simulink model "elevatorMod"  (R2020a)
settings: Solver=VariableStepAuto  StartTime=0.0  StopTime=inf  RelTol=1e-3
PreLoadFcn:
  | slplc.api.loadDataTypes;
undefined symbols (not defined in the file): BOOL, DINT, INT, slplc
libraries: simulink x1
(part 28 of 39)

== system elevatorMod/PLCControllerSuite/__Logic/Task/Program/__Logic/XIC3/Instruction_Enable/__CoreVarRead ==
  DataRead : DataStoreRead  DataStoreName=xxx_PLC_VAR_F1PB
  y : Outport  VectorParamsAs1DForOutWhenUnconnected=off
  wires:
  DataRead/1 -> y/1

== system elevatorMod/PLCControllerSuite/__Logic/Task/Program/__Logic/XIC3/RungInOverride/ForceRungInFalseRead ==
  __CoreLabelRead : Subsystem  Tag=CoreVarReadBlock  DisableCoverage=on  TreatAsAtomicUnit=on  mask{PLCBlockType=CoreLabelRead}
      mask init:
      | slplc.callbacks.initRoutineLabelRead(gcb);
      mask Help: web([docroot '/plccoder/ref/__corelabelread' '.html']);
      mask DialogControl PLCBlockTitle Prompt: Core Label Read
  Out1 : Outport  VectorParamsAs1DForOutWhenUnconnected=off
  wires:
  __CoreLabelRead/1(Out1) -> Out1/1

== system elevatorMod/PLCControllerSuite/__Logic/Task/Program/__Logic/XIC30/BlockEnableRead/__CoreLabelRead ==
  DataRead : DataStoreRead  DataStoreName=x_PLCLabel__s4_3653__Block_Enable
  Out1 : Outport  VectorParamsAs1DForOutWhenUnconnected=off
  wires:
  DataRead/1 -> Out1/1

== system elevatorMod/PLCControllerSuite/__Logic/Task/Program/__Logic/XIC30/Instruction_Enable/__CoreVarRead ==
  DataRead : DataStoreRead  DataStoreName=xxx_PLC_VAR_F1PBHold
  y : Outport  VectorParamsAs1DForOutWhenUnconnected=off
  wires:
  DataRead/1 -> y/1

== system elevatorMod/PLCControllerSuite/__Logic/Task/Program/__Logic/XIC30/RungInOverride/ForceRungInFalseRead ==
  __CoreLabelRead : Subsystem  Tag=CoreVarReadBlock  DisableCoverage=on  TreatAsAtomicUnit=on  mask{PLCBlockType=CoreLabelRead}
      mask init:
      | slplc.callbacks.initRoutineLabelRead(gcb);
      mask Help: web([docroot '/plccoder/ref/__corelabelread' '.html']);
      mask DialogControl PLCBlockTitle Prompt: Core Label Read
  Out1 : Outport  VectorParamsAs1DForOutWhenUnconnected=off
  wires:
  __CoreLabelRead/1(Out1) -> Out1/1

== system elevatorMod/PLCControllerSuite/__Logic/Task/Program/__Logic/XIC31/BlockEnableRead/__CoreLabelRead ==
  DataRead : DataStoreRead  DataStoreName=x_PLCLabel__s4_3653__Block_Enable
  Out1 : Outport  VectorParamsAs1DForOutWhenUnconnected=off
  wires:
  DataRead/1 -> Out1/1

== system elevatorMod/PLCControllerSuite/__Logic/Task/Program/__Logic/XIC31/Instruction_Enable/__CoreVarRead ==
  DataRead : DataStoreRead  DataStoreName=xxx_PLC_VAR_StartHold
  y : Outport  VectorParamsAs1DForOutWhenUnconnected=off
  wires:
  DataRead/1 -> y/1

== system elevatorMod/PLCControllerSuite/__Logic/Task/Program/__Logic/XIC31/RungInOverride/ForceRungInFalseRead ==
  __CoreLabelRead : Subsystem  Tag=CoreVarReadBlock  DisableCoverage=on  TreatAsAtomicUnit=on  mask{PLCBlockType=CoreLabelRead}
      mask init:
      | slplc.callbacks.initRoutineLabelRead(gcb);
      mask Help: web([docroot '/plccoder/ref/__corelabelread' '.html']);
      mask DialogControl PLCBlockTitle Prompt: Core Label Read
  Out1 : Outport  VectorParamsAs1DForOutWhenUnconnected=off
  wires:
  __CoreLabelRead/1(Out1) -> Out1/1

== system elevatorMod/PLCControllerSuite/__Logic/Task/Program/__Logic/XIC32/BlockEnableRead/__CoreLabelRead ==
  DataRead : DataStoreRead  DataStoreName=x_PLCLabel__s4_3653__Block_Enable
  Out1 : Outport  VectorParamsAs1DForOutWhenUnconnected=off
  wires:
  DataRead/1 -> Out1/1

== system elevatorMod/PLCControllerSuite/__Logic/Task/Program/__Logic/XIC32/Instruction_Enable/__CoreVarRead ==
  DataRead : DataStoreRead  DataStoreName=xxx_PLC_VAR_LSTDIRUP
  y : Outport  VectorParamsAs1DForOutWhenUnconnected=off
  wires:
  DataRead/1 -> y/1

== system elevatorMod/PLCControllerSuite/__Logic/Task/Program/__Logic/XIC32/RungInOverride/ForceRungInFalseRead ==
  __CoreLabelRead : Subsystem  Tag=CoreVarReadBlock  DisableCoverage=on  TreatAsAtomicUnit=on  mask{PLCBlockType=CoreLabelRead}
      mask init:
      | slplc.callbacks.initRoutineLabelRead(gcb);
      mask Help: web([docroot '/plccoder/ref/__corelabelread' '.html']);
      mask DialogControl PLCBlockTitle Prompt: Core Label Read
  Out1 : Outport  VectorParamsAs1DForOutWhenUnconnected=off
  wires:
  __CoreLabelRead/1(Out1) -> Out1/1

== system elevatorMod/PLCControllerSuite/__Logic/Task/Program/__Logic/XIC33/BlockEnableRead/__CoreLabelRead ==
  DataRead : DataStoreRead  DataStoreName=x_PLCLabel__s4_3653__Block_Enable
  Out1 : Outport  VectorParamsAs1DForOutWhenUnconnected=off
  wires:
  DataRead/1 -> Out1/1

== system elevatorMod/PLCControllerSuite/__Logic/Task/Program/__Logic/XIC33/Instruction_Enable/__CoreVarRead ==
  DataRead : DataStoreRead  DataStoreName=xxx_PLC_VAR_GOINGUP
  y : Outport  VectorParamsAs1DForOutWhenUnconnected=off
  wires:
  DataRead/1 -> y/1

== system elevatorMod/PLCControllerSuite/__Logic/Task/Program/__Logic/XIC33/RungInOverride/ForceRungInFalseRead ==
  __CoreLabelRead : Subsystem  Tag=CoreVarReadBlock  DisableCoverage=on  TreatAsAtomicUnit=on  mask{PLCBlockType=CoreLabelRead}
      mask init:
      | slplc.callbacks.initRoutineLabelRead(gcb);
      mask Help: web([docroot '/plccoder/ref/__corelabelread' '.html']);
      mask DialogControl PLCBlockTitle Prompt: Core Label Read
  Out1 : Outport  VectorParamsAs1DForOutWhenUnconnected=off
  wires:
  __CoreLabelRead/1(Out1) -> Out1/1

== system elevatorMod/PLCControllerSuite/__Logic/Task/Program/__Logic/XIC34/BlockEnableRead/__CoreLabelRead ==
  DataRead : DataStoreRead  DataStoreName=x_PLCLabel__s4_3653__Block_Enable
  Out1 : Outport  VectorParamsAs1DForOutWhenUnconnected=off
  wires:
  DataRead/1 -> Out1/1

== system elevatorMod/PLCControllerSuite/__Logic/Task/Program/__Logic/XIC34/Instruction_Enable/__CoreVarRead ==
  DataRead : DataStoreRead  DataStoreName=xxx_PLC_VAR_MTRON
  y : Outport  VectorParamsAs1DForOutWhenUnconnected=off
  wires:
  DataRead/1 -> y/1

== system elevatorMod/PLCControllerSuite/__Logic/Task/Program/__Logic/XIC34/RungInOverride/ForceRungInFalseRead ==
  __CoreLabelRead : Subsystem  Tag=CoreVarReadBlock  DisableCoverage=on  TreatAsAtomicUnit=on  mask{PLCBlockType=CoreLabelRead}
      mask init:
      | slplc.callbacks.initRoutineLabelRead(gcb);
      mask Help: web([docroot '/plccoder/ref/__corelabelread' '.html']);
      mask DialogControl PLCBlockTitle Prompt: Core Label Read
  Out1 : Outport  VectorParamsAs1DForOutWhenUnconnected=off
  wires:
  __CoreLabelRead/1(Out1) -> Out1/1

== system elevatorMod/PLCControllerSuite/__Logic/Task/Program/__Logic/XIC35/BlockEnableRead/__CoreLabelRead ==
  DataRead : DataStoreRead  DataStoreName=x_PLCLabel__s4_3653__Block_Enable
  Out1 : Outport  VectorParamsAs1DForOutWhenUnconnected=off
  wires:
  DataRead/1 -> Out1/1

== system elevatorMod/PLCControllerSuite/__Logic/Task/Program/__Logic/XIC35/Instruction_Enable/__CoreVarRead ==
  DataRead : DataStoreRead  DataStoreName=xxx_PLC_VAR_F2PBHold
  y : Outport  VectorParamsAs1DForOutWhenUnconnected=off
  wires:
  DataRead/1 -> y/1

== system elevatorMod/PLCControllerSuite/__Logic/Task/Program/__Logic/XIC35/RungInOverride/ForceRungInFalseRead ==
  __CoreLabelRead : Subsystem  Tag=CoreVarReadBlock  DisableCoverage=on  TreatAsAtomicUnit=on  mask{PLCBlockType=CoreLabelRead}
      mask init:
      | slplc.callbacks.initRoutineLabelRead(gcb);
      mask Help: web([docroot '/plccoder/ref/__corelabelread' '.html']);
      mask DialogControl PLCBlockTitle Prompt: Core Label Read
  Out1 : Outport  VectorParamsAs1DForOutWhenUnconnected=off
  wires:
  __CoreLabelRead/1(Out1) -> Out1/1

== system elevatorMod/PLCControllerSuite/__Logic/Task/Program/__Logic/XIC36/BlockEnableRead/__CoreLabelRead ==
  DataRead : DataStoreRead  DataStoreName=x_PLCLabel__s4_3653__Block_Enable
  Out1 : Outport  VectorParamsAs1DForOutWhenUnconnected=off
  wires:
  DataRead/1 -> Out1/1

== system elevatorMod/PLCControllerSuite/__Logic/Task/Program/__Logic/XIC36/Instruction_Enable/__CoreVarRead ==
  DataRead : DataStoreRead  DataStoreName=xxx_PLC_VAR_F3DownBHold
  y : Outport  VectorParamsAs1DForOutWhenUnconnected=off
  wires:
  DataRead/1 -> y/1

== system elevatorMod/PLCControllerSuite/__Logic/Task/Program/__Logic/XIC36/RungInOverride/ForceRungInFalseRead ==
  __CoreLabelRead : Subsystem  Tag=CoreVarReadBlock  DisableCoverage=on  TreatAsAtomicUnit=on  mask{PLCBlockType=CoreLabelRead}
      mask init:
      | slplc.callbacks.initRoutineLabelRead(gcb);
      mask Help: web([docroot '/plccoder/ref/__corelabelread' '.html']);
      mask DialogControl PLCBlockTitle Prompt: Core Label Read
  Out1 : Outport  VectorParamsAs1DForOutWhenUnconnected=off
  wires:
  __CoreLabelRead/1(Out1) -> Out1/1

== system elevatorMod/PLCControllerSuite/__Logic/Task/Program/__Logic/XIC37/BlockEnableRead/__CoreLabelRead ==
  DataRead : DataStoreRead  DataStoreName=x_PLCLabel__s4_3653__Block_Enable
  Out1 : Outport  VectorParamsAs1DForOutWhenUnconnected=off
  wires:
  DataRead/1 -> Out1/1

== system elevatorMod/PLCControllerSuite/__Logic/Task/Program/__Logic/XIC37/Instruction_Enable/__CoreVarRead ==
  DataRead : DataStoreRead  DataStoreName=xxx_PLC_VAR_F2PBHold
  y : Outport  VectorParamsAs1DForOutWhenUnconnected=off
  wires:
  DataRead/1 -> y/1

== system elevatorMod/PLCControllerSuite/__Logic/Task/Program/__Logic/XIC37/RungInOverride/ForceRungInFalseRead ==
  __CoreLabelRead : Subsystem  Tag=CoreVarReadBlock  DisableCoverage=on  TreatAsAtomicUnit=on  mask{PLCBlockType=CoreLabelRead}
      mask init:
      | slplc.callbacks.initRoutineLabelRead(gcb);
      mask Help: web([docroot '/plccoder/ref/__corelabelread' '.html']);
      mask DialogControl PLCBlockTitle Prompt: Core Label Read
  Out1 : Outport  VectorParamsAs1DForOutWhenUnconnected=off
  wires:
  __CoreLabelRead/1(Out1) -> Out1/1

== system elevatorMod/PLCControllerSuite/__Logic/Task/Program/__Logic/XIC38/BlockEnableRead/__CoreLabelRead ==
  DataRead : DataStoreRead  DataStoreName=x_PLCLabel__s4_3653__Block_Enable
  Out1 : Outport  VectorParamsAs1DForOutWhenUnconnected=off
  wires:
  DataRead/1 -> Out1/1

== system elevatorMod/PLCControllerSuite/__Logic/Task/Program/__Logic/XIC38/Instruction_Enable/__CoreVarRead ==
  DataRead : DataStoreRead  DataStoreName=xxx_PLC_VAR_MTRON
  y : Outport  VectorParamsAs1DForOutWhenUnconnected=off
  wires:
  DataRead/1 -> y/1

== system elevatorMod/PLCControllerSuite/__Logic/Task/Program/__Logic/XIC38/RungInOverride/ForceRungInFalseRead ==
  __CoreLabelRead : Subsystem  Tag=CoreVarReadBlock  DisableCoverage=on  TreatAsAtomicUnit=on  mask{PLCBlockType=CoreLabelRead}
      mask init:
      | slplc.callbacks.initRoutineLabelRead(gcb);
      mask Help: web([docroot '/plccoder/ref/__corelabelread' '.html']);
      mask DialogControl PLCBlockTitle Prompt: Core Label Read
  Out1 : Outport  VectorParamsAs1DForOutWhenUnconnected=off
  wires:
  __CoreLabelRead/1(Out1) -> Out1/1

== system elevatorMod/PLCControllerSuite/__Logic/Task/Program/__Logic/XIC39/BlockEnableRead/__CoreLabelRead ==
  DataRead : DataStoreRead  DataStoreName=x_PLCLabel__s4_3653__Block_Enable
  Out1 : Outport  VectorParamsAs1DForOutWhenUnconnected=off
  wires:
  DataRead/1 -> Out1/1

== system elevatorMod/PLCControllerSuite/__Logic/Task/Program/__Logic/XIC39/Instruction_Enable/__CoreVarRead ==
  DataRead : DataStoreRead  DataStoreName=xxx_PLC_VAR_RMPUPTRG
  y : Outport  VectorParamsAs1DForOutWhenUnconnected=off
  wires:
  DataRead/1 -> y/1

== system elevatorMod/PLCControllerSuite/__Logic/Task/Program/__Logic/XIC39/RungInOverride/ForceRungInFalseRead ==
  __CoreLabelRead : Subsystem  Tag=CoreVarReadBlock  DisableCoverage=on  TreatAsAtomicUnit=on  mask{PLCBlockType=CoreLabelRead}
      mask init:
      | slplc.callbacks.initRoutineLabelRead(gcb);
      mask Help: web([docroot '/plccoder/ref/__corelabelread' '.html']);
      mask DialogControl PLCBlockTitle Prompt: Core Label Read
  Out1 : Outport  VectorParamsAs1DForOutWhenUnconnected=off
  wires:
  __CoreLabelRead/1(Out1) -> Out1/1

== system elevatorMod/PLCControllerSuite/__Logic/Task/Program/__Logic/XIC4/BlockEnableRead/__CoreLabelRead ==
  DataRead : DataStoreRead  DataStoreName=x_PLCLabel__s4_3653__Block_Enable
  Out1 : Outport  VectorParamsAs1DForOutWhenUnconnected=off
  wires:
  DataRead/1 -> Out1/1

== system elevatorMod/PLCControllerSuite/__Logic/Task/Program/__Logic/XIC4/Instruction_Enable/__CoreVarRead ==
  DataRead : DataStoreRead  DataStoreName=xxx_PLC_VAR_F1PBHold
  y : Outport  VectorParamsAs1DForOutWhenUnconnected=off
  wires:
  DataRead/1 -> y/1

== system elevatorMod/PLCControllerSuite/__Logic/Task/Program/__Logic/XIC4/RungInOverride/ForceRungInFalseRead ==
  __CoreLabelRead : Subsystem  Tag=CoreVarReadBlock  DisableCoverage=on  TreatAsAtomicUnit=on  mask{PLCBlockType=CoreLabelRead}
      mask init:
      | slplc.callbacks.initRoutineLabelRead(gcb);
      mask Help: web([docroot '/plccoder/ref/__corelabelread' '.html']);
      mask DialogControl PLCBlockTitle Prompt: Core Label Read
  Out1 : Outport  VectorParamsAs1DForOutWhenUnconnected=off
  wires:
  __CoreLabelRead/1(Out1) -> Out1/1

== system elevatorMod/PLCControllerSuite/__Logic/Task/Program/__Logic/XIC40/BlockEnableRead/__CoreLabelRead ==
  DataRead : DataStoreRead  DataStoreName=x_PLCLabel__s4_3653__Block_Enable
  Out1 : Outport  VectorParamsAs1DForOutWhenUnconnected=off
  wires:
  DataRead/1 -> Out1/1

== system elevatorMod/PLCControllerSuite/__Logic/Task/Program/__Logic/XIC40/Instruction_Enable/__CoreVarRead ==
  DataRead : DataStoreRead  DataStoreName=xxx_PLC_VAR_RMPUP
  y : Outport  VectorParamsAs1DForOutWhenUnconnected=off
  wires:
  DataRead/1 -> y/1

== system elevatorMod/PLCControllerSuite/__Logic/Task/Program/__Logic/XIC40/RungInOverride/ForceRungInFalseRead ==
  __CoreLabelRead : Subsystem  Tag=CoreVarReadBlock  DisableCoverage=on  TreatAsAtomicUnit=on  mask{PLCBlockType=CoreLabelRead}
      mask init:
      | slplc.callbacks.initRoutineLabelRead(gcb);
      mask Help: web([docroot '/plccoder/ref/__corelabelread' '.html']);
      mask DialogControl PLCBlockTitle Prompt: Core Label Read
  Out1 : Outport  VectorParamsAs1DForOutWhenUnconnected=off
  wires:
  __CoreLabelRead/1(Out1) -> Out1/1

== system elevatorMod/PLCControllerSuite/__Logic/Task/Program/__Logic/XIC41/BlockEnableRead/__CoreLabelRead ==
  DataRead : DataStoreRead  DataStoreName=x_PLCLabel__s4_3653__Block_Enable
  Out1 : Outport  VectorParamsAs1DForOutWhenUnconnected=off
  wires:
  DataRead/1 -> Out1/1

== system elevatorMod/PLCControllerSuite/__Logic/Task/Program/__Logic/XIC41/Instruction_Enable/__CoreVarRead ==
  DataRead : DataStoreRead  DataStoreName=xxx_PLC_VAR_SENCHK
  y : Outport  VectorParamsAs1DForOutWhenUnconnected=off
  wires:
  DataRead/1 -> y/1

== system elevatorMod/PLCControllerSuite/__Logic/Task/Program/__Logic/XIC41/RungInOverride/ForceRungInFalseRead ==
  __CoreLabelRead : Subsystem  Tag=CoreVarReadBlock  DisableCoverage=on  TreatAsAtomicUnit=on  mask{PLCBlockType=CoreLabelRead}
      mask init:
      | slplc.callbacks.initRoutineLabelRead(gcb);
      mask Help: web([docroot '/plccoder/ref/__corelabelread' '.html']);
      mask DialogControl PLCBlockTitle Prompt: Core Label Read
  Out1 : Outport  VectorParamsAs1DForOutWhenUnconnected=off
  wires:
  __CoreLabelRead/1(Out1) -> Out1/1

== system elevatorMod/PLCControllerSuite/__Logic/Task/Program/__Logic/XIC42/BlockEnableRead/__CoreLabelRead ==
  DataRead : DataStoreRead  DataStoreName=x_PLCLabel__s4_3653__Block_Enable
  Out1 : Outport  VectorParamsAs1DForOutWhenUnconnected=off
  wires:
  DataRead/1 -> Out1/1

== system elevatorMod/PLCControllerSuite/__Logic/Task/Program/__Logic/XIC42/Instruction_Enable/__CoreVarRead ==
  DataRead : DataStoreRead  DataStoreName=xxx_PLC_VAR_StartHold
  y : Outport  VectorParamsAs1DForOutWhenUnconnected=off
  wires:
  DataRead/1 -> y/1

== system elevatorMod/PLCControllerSuite/__Logic/Task/Program/__Logic/XIC42/RungInOverride/ForceRungInFalseRead ==
  __CoreLabelRead : Subsystem  Tag=CoreVarReadBlock  DisableCoverage=on  TreatAsAtomicUnit=on  mask{PLCBlockType=CoreLabelRead}
      mask init:
      | slplc.callbacks.initRoutineLabelRead(gcb);
      mask Help: web([docroot '/plccoder/ref/__corelabelread' '.html']);
      mask DialogControl PLCBlockTitle Prompt: Core Label Read
  Out1 : Outport  VectorParamsAs1DForOutWhenUnconnected=off
  wires:
  __CoreLabelRead/1(Out1) -> Out1/1

== system elevatorMod/PLCControllerSuite/__Logic/Task/Program/__Logic/XIC43/BlockEnableRead/__CoreLabelRead ==
  DataRead : DataStoreRead  DataStoreName=x_PLCLabel__s4_3653__Block_Enable
  Out1 : Outport  VectorParamsAs1DForOutWhenUnconnected=off
  wires:
  DataRead/1 -> Out1/1

== system elevatorMod/PLCControllerSuite/__Logic/Task/Program/__Logic/XIC43/Instruction_Enable/__CoreVarRead ==
  DataRead : DataStoreRead  DataStoreName=xxx_PLC_VAR_TempS3LUp
  y : Outport  VectorParamsAs1DForOutWhenUnconnected=off
  wires:
  DataRead/1 -> y/1

== system elevatorMod/PLCControllerSuite/__Logic/Task/Program/__Logic/XIC43/RungInOverride/ForceRungInFalseRead ==
  __CoreLabelRead : Subsystem  Tag=CoreVarReadBlock  DisableCoverage=on  TreatAsAtomicUnit=on  mask{PLCBlockType=CoreLabelRead}
      mask init:
      | slplc.callbacks.initRoutineLabelRead(gcb);
      mask Help: web([docroot '/plccoder/ref/__corelabelread' '.html']);
      mask DialogControl PLCBlockTitle Prompt: Core Label Read
  Out1 : Outport  VectorParamsAs1DForOutWhenUnconnected=off
  wires:
  __CoreLabelRead/1(Out1) -> Out1/1

== system elevatorMod/PLCControllerSuite/__Logic/Task/Program/__Logic/XIC44/BlockEnableRead/__CoreLabelRead ==
  DataRead : DataStoreRead  DataStoreName=x_PLCLabel__s4_3653__Block_Enable
  Out1 : Outport  VectorParamsAs1DForOutWhenUnconnected=off
  wires:
  DataRead/1 -> Out1/1

== system elevatorMod/PLCControllerSuite/__Logic/Task/Program/__Logic/XIC44/Instruction_Enable/__CoreVarRead ==
  DataRead : DataStoreRead  DataStoreName=xxx_PLC_VAR_MemoryGoUp
  y : Outport  VectorParamsAs1DForOutWhenUnconnected=off
  wires:
  DataRead/1 -> y/1

== system elevatorMod/PLCControllerSuite/__Logic/Task/Program/__Logic/XIC44/RungInOverride/ForceRungInFalseRead ==
  __CoreLabelRead : Subsystem  Tag=CoreVarReadBlock  DisableCoverage=on  TreatAsAtomicUnit=on  mask{PLCBlockType=CoreLabelRead}
      mask init:
      | slplc.callbacks.initRoutineLabelRead(gcb);
      mask Help: web([docroot '/plccoder/ref/__corelabelread' '.html']);
      mask DialogControl PLCBlockTitle Prompt: Core Label Read
  Out1 : Outport  VectorParamsAs1DForOutWhenUnconnected=off
  wires:
  __CoreLabelRead/1(Out1) -> Out1/1

== system elevatorMod/PLCControllerSuite/__Logic/Task/Program/__Logic/XIC45/BlockEnableRead/__CoreLabelRead ==
  DataRead : DataStoreRead  DataStoreName=x_PLCLabel__s4_3653__Block_Enable
  Out1 : Outport  VectorParamsAs1DForOutWhenUnconnected=off
  wires:
  DataRead/1 -> Out1/1

== system elevatorMod/PLCControllerSuite/__Logic/Task/Program/__Logic/XIC45/Instruction_Enable/__CoreVarRead ==
  DataRead : DataStoreRead  DataStoreName=xxx_PLC_VAR_StartHold
  y : Outport  VectorParamsAs1DForOutWhenUnconnected=off
  wires:
  DataRead/1 -> y/1

== system elevatorMod/PLCControllerSuite/__Logic/Task/Program/__Logic/XIC45/RungInOverride/ForceRungInFalseRead ==
  __CoreLabelRead : Subsystem  Tag=CoreVarReadBlock  DisableCoverage=on  TreatAsAtomicUnit=on  mask{PLCBlockType=CoreLabelRead}
      mask init:
      | slplc.callbacks.initRoutineLabelRead(gcb);
      mask Help: web([docroot '/plccoder/ref/__corelabelread' '.html']);
      mask DialogControl PLCBlockTitle Prompt: Core Label Read
  Out1 : Outport  VectorParamsAs1DForOutWhenUnconnected=off
  wires:
  __CoreLabelRead/1(Out1) -> Out1/1

== system elevatorMod/PLCControllerSuite/__Logic/Task/Program/__Logic/XIC46/BlockEnableRead/__CoreLabelRead ==
  DataRead : DataStoreRead  DataStoreName=x_PLCLabel__s4_3653__Block_Enable
  Out1 : Outport  VectorParamsAs1DForOutWhenUnconnected=off
  wires:
  DataRead/1 -> Out1/1

== system elevatorMod/PLCControllerSuite/__Logic/Task/Program/__Logic/XIC46/Instruction_Enable/__CoreVarRead ==
  DataRead : DataStoreRead  DataStoreName=xxx_PLC_VAR_S1H
  y : Outport  VectorParamsAs1DForOutWhenUnconnected=off
  wires:
  DataRead/1 -> y/1

== system elevatorMod/PLCControllerSuite/__Logic/Task/Program/__Logic/XIC46/RungInOverride/ForceRungInFalseRead ==
  __CoreLabelRead : Subsystem  Tag=CoreVarReadBlock  DisableCoverage=on  TreatAsAtomicUnit=on  mask{PLCBlockType=CoreLabelRead}
      mask init:
      | slplc.callbacks.initRoutineLabelRead(gcb);
      mask Help: web([docroot '/plccoder/ref/__corelabelread' '.html']);
      mask DialogControl PLCBlockTitle Prompt: Core Label Read
  Out1 : Outport  VectorParamsAs1DForOutWhenUnconnected=off
  wires:
  __CoreLabelRead/1(Out1) -> Out1/1

== system elevatorMod/PLCControllerSuite/__Logic/Task/Program/__Logic/XIC47/BlockEnableRead/__CoreLabelRead ==
  DataRead : DataStoreRead  DataStoreName=x_PLCLabel__s4_3653__Block_Enable
  Out1 : Outport  VectorParamsAs1DForOutWhenUnconnected=off
  wires:
  DataRead/1 -> Out1/1

== system elevatorMod/PLCControllerSuite/__Logic/Task/Program/__Logic/XIC47/Instruction_Enable/__CoreVarRead ==
  DataRead : DataStoreRead  DataStoreName=xxx_PLC_VAR_S2L
  y : Outport  VectorParamsAs1DForOutWhenUnconnected=off
  wires:
  DataRead/1 -> y/1

== system elevatorMod/PLCControllerSuite/__Logic/Task/Program/__Logic/XIC47/RungInOverride/ForceRungInFalseRead ==
  __CoreLabelRead : Subsystem  Tag=CoreVarReadBlock  DisableCoverage=on  TreatAsAtomicUnit=on  mask{PLCBlockType=CoreLabelRead}
      mask init:
      | slplc.callbacks.initRoutineLabelRead(gcb);
      mask Help: web([docroot '/plccoder/ref/__corelabelread' '.html']);
      mask DialogControl PLCBlockTitle Prompt: Core Label Read
  Out1 : Outport  VectorParamsAs1DForOutWhenUnconnected=off
  wires:
  __CoreLabelRead/1(Out1) -> Out1/1

== system elevatorMod/PLCControllerSuite/__Logic/Task/Program/__Logic/XIC48/BlockEnableRead/__CoreLabelRead ==
  DataRead : DataStoreRead  DataStoreName=x_PLCLabel__s4_3653__Block_Enable
  Out1 : Outport  VectorParamsAs1DForOutWhenUnconnected=off
  wires:
  DataRead/1 -> Out1/1

== system elevatorMod/PLCControllerSuite/__Logic/Task/Program/__Logic/XIC48/Instruction_Enable/__CoreVarRead ==
  DataRead : DataStoreRead  DataStoreName=xxx_PLC_VAR_F2UpDownBHold
  y : Outport  VectorParamsAs1DForOutWhenUnconnected=off
  wires:
  DataRead/1 -> y/1

== system elevatorMod/PLCControllerSuite/__Logic/Task/Program/__Logic/XIC48/RungInOverride/ForceRungInFalseRead ==
  __CoreLabelRead : Subsystem  Tag=CoreVarReadBlock  DisableCoverage=on  TreatAsAtomicUnit=on  mask{PLCBlockType=CoreLabelRead}
      mask init:
      | slplc.callbacks.initRoutineLabelRead(gcb);
      mask Help: web([docroot '/plccoder/ref/__corelabelread' '.html']);
      mask DialogControl PLCBlockTitle Prompt: Core Label Read
  Out1 : Outport  VectorParamsAs1DForOutWhenUnconnected=off
  wires:
  __CoreLabelRead/1(Out1) -> Out1/1

== system elevatorMod/PLCControllerSuite/__Logic/Task/Program/__Logic/XIC49/BlockEnableRead/__CoreLabelRead ==
  DataRead : DataStoreRead  DataStoreName=x_PLCLabel__s4_3653__Block_Enable
  Out1 : Outport  VectorParamsAs1DForOutWhenUnconnected=off
  wires:
  DataRead/1 -> Out1/1

== system elevatorMod/PLCControllerSuite/__Logic/Task/Program/__Logic/XIC49/Instruction_Enable/__CoreVarRead ==
  DataRead : DataStoreRead  DataStoreName=xxx_PLC_VAR_S3L
  y : Outport  VectorParamsAs1DForOutWhenUnconnected=off
  wires:
  DataRead/1 -> y/1

== system elevatorMod/PLCControllerSuite/__Logic/Task/Program/__Logic/XIC49/RungInOverride/ForceRungInFalseRead ==
  __CoreLabelRead : Subsystem  Tag=CoreVarReadBlock  DisableCoverage=on  TreatAsAtomicUnit=on  mask{PLCBlockType=CoreLabelRead}
      mask init:
      | slplc.callbacks.initRoutineLabelRead(gcb);
      mask Help: web([docroot '/plccoder/ref/__corelabelread' '.html']);
      mask DialogControl PLCBlockTitle Prompt: Core Label Read
  Out1 : Outport  VectorParamsAs1DForOutWhenUnconnected=off
  wires:
  __CoreLabelRead/1(Out1) -> Out1/1

== system elevatorMod/PLCControllerSuite/__Logic/Task/Program/__Logic/XIC5/BlockEnableRead/__CoreLabelRead ==
  DataRead : DataStoreRead  DataStoreName=x_PLCLabel__s4_3653__Block_Enable
  Out1 : Outport  VectorParamsAs1DForOutWhenUnconnected=off
  wires:
  DataRead/1 -> Out1/1

== system elevatorMod/PLCControllerSuite/__Logic/Task/Program/__Logic/XIC5/Instruction_Enable/__CoreVarRead ==
  DataRead : DataStoreRead  DataStoreName=xxx_PLC_VAR_StartHold
  y : Outport  VectorParamsAs1DForOutWhenUnconnected=off
  wires:
  DataRead/1 -> y/1

== system elevatorMod/PLCControllerSuite/__Logic/Task/Program/__Logic/XIC5/RungInOverride/ForceRungInFalseRead ==
  __CoreLabelRead : Subsystem  Tag=CoreVarReadBlock  DisableCoverage=on  TreatAsAtomicUnit=on  mask{PLCBlockType=CoreLabelRead}
      mask init:
      | slplc.callbacks.initRoutineLabelRead(gcb);
      mask Help: web([docroot '/plccoder/ref/__corelabelread' '.html']);
      mask DialogControl PLCBlockTitle Prompt: Core Label Read
  Out1 : Outport  VectorParamsAs1DForOutWhenUnconnected=off
  wires:
  __CoreLabelRead/1(Out1) -> Out1/1

== system elevatorMod/PLCControllerSuite/__Logic/Task/Program/__Logic/XIC50/BlockEnableRead/__CoreLabelRead ==
  DataRead : DataStoreRead  DataStoreName=x_PLCLabel__s4_3653__Block_Enable
  Out1 : Outport  VectorParamsAs1DForOutWhenUnconnected=off
  wires:
  DataRead/1 -> Out1/1

== system elevatorMod/PLCControllerSuite/__Logic/Task/Program/__Logic/XIC50/Instruction_Enable/__CoreVarRead ==
  DataRead : DataStoreRead  DataStoreName=xxx_PLC_VAR_S2H
  y : Outport  VectorParamsAs1DForOutWhenUnconnected=off
  wires:
  DataRead/1 -> y/1

== system elevatorMod/PLCControllerSuite/__Logic/Task/Program/__Logic/XIC50/RungInOverride/ForceRungInFalseRead ==
  __CoreLabelRead : Subsystem  Tag=CoreVarReadBlock  DisableCoverage=on  TreatAsAtomicUnit=on  mask{PLCBlockType=CoreLabelRead}
      mask init:
      | slplc.callbacks.initRoutineLabelRead(gcb);
      mask Help: web([docroot '/plccoder/ref/__corelabelread' '.html']);
      mask DialogControl PLCBlockTitle Prompt: Core Label Read
  Out1 : Outport  VectorParamsAs1DForOutWhenUnconnected=off
  wires:
  __CoreLabelRead/1(Out1) -> Out1/1

== system elevatorMod/PLCControllerSuite/__Logic/Task/Program/__Logic/XIC51/BlockEnableRead/__CoreLabelRead ==
  DataRead : DataStoreRead  DataStoreName=x_PLCLabel__s4_3653__Block_Enable
  Out1 : Outport  VectorParamsAs1DForOutWhenUnconnected=off
  wires:
  DataRead/1 -> Out1/1

== system elevatorMod/PLCControllerSuite/__Logic/Task/Program/__Logic/XIC51/Instruction_Enable/__CoreVarRead ==
  DataRead : DataStoreRead  DataStoreName=xxx_PLC_VAR_F1PBHold
  y : Outport  VectorParamsAs1DForOutWhenUnconnected=off
  wires:
  DataRead/1 -> y/1

== system elevatorMod/PLCControllerSuite/__Logic/Task/Program/__Logic/XIC51/RungInOverride/ForceRungInFalseRead ==
  __CoreLabelRead : Subsystem  Tag=CoreVarReadBlock  DisableCoverage=on  TreatAsAtomicUnit=on  mask{PLCBlockType=CoreLabelRead}
      mask init:
      | slplc.callbacks.initRoutineLabelRead(gcb);
      mask Help: web([docroot '/plccoder/ref/__corelabelread' '.html']);
      mask DialogControl PLCBlockTitle Prompt: Core Label Read
  Out1 : Outport  VectorParamsAs1DForOutWhenUnconnected=off
  wires:
  __CoreLabelRead/1(Out1) -> Out1/1

== system elevatorMod/PLCControllerSuite/__Logic/Task/Program/__Logic/XIC52/BlockEnableRead/__CoreLabelRead ==
  DataRead : DataStoreRead  DataStoreName=x_PLCLabel__s4_3653__Block_Enable
  Out1 : Outport  VectorParamsAs1DForOutWhenUnconnected=off
  wires:
  DataRead/1 -> Out1/1

== system elevatorMod/PLCControllerSuite/__Logic/Task/Program/__Logic/XIC52/Instruction_Enable/__CoreVarRead ==
  DataRead : DataStoreRead  DataStoreName=xxx_PLC_VAR_F2UpDownBHold
  y : Outport  VectorParamsAs1DForOutWhenUnconnected=off
  wires:
  DataRead/1 -> y/1

== system elevatorMod/PLCControllerSuite/__Logic/Task/Program/__Logic/XIC52/RungInOverride/ForceRungInFalseRead ==
  __CoreLabelRead : Subsystem  Tag=CoreVarReadBlock  DisableCoverage=on  TreatAsAtomicUnit=on  mask{PLCBlockType=CoreLabelRead}
      mask init:
      | slplc.callbacks.initRoutineLabelRead(gcb);
      mask Help: web([docroot '/plccoder/ref/__corelabelread' '.html']);
      mask DialogControl PLCBlockTitle Prompt: Core Label Read
  Out1 : Outport  VectorParamsAs1DForOutWhenUnconnected=off
  wires:
  __CoreLabelRead/1(Out1) -> Out1/1

== system elevatorMod/PLCControllerSuite/__Logic/Task/Program/__Logic/XIC53/BlockEnableRead/__CoreLabelRead ==
  DataRead : DataStoreRead  DataStoreName=x_PLCLabel__s4_3653__Block_Enable
  Out1 : Outport  VectorParamsAs1DForOutWhenUnconnected=off
  wires:
  DataRead/1 -> Out1/1

== system elevatorMod/PLCControllerSuite/__Logic/Task/Program/__Logic/XIC53/Instruction_Enable/__CoreVarRead ==
  DataRead : DataStoreRead  DataStoreName=xxx_PLC_VAR_GOINGUP
  y : Outport  VectorParamsAs1DForOutWhenUnconnected=off
  wires:
  DataRead/1 -> y/1

== system elevatorMod/PLCControllerSuite/__Logic/Task/Program/__Logic/XIC53/RungInOverride/ForceRungInFalseRead ==
  __CoreLabelRead : Subsystem  Tag=CoreVarReadBlock  DisableCoverage=on  TreatAsAtomicUnit=on  mask{PLCBlockType=CoreLabelRead}
      mask init:
      | slplc.callbacks.initRoutineLabelRead(gcb);
      mask Help: web([docroot '/plccoder/ref/__corelabelread' '.html']);
      mask DialogControl PLCBlockTitle Prompt: Core Label Read
  Out1 : Outport  VectorParamsAs1DForOutWhenUnconnected=off
  wires:
  __CoreLabelRead/1(Out1) -> Out1/1

== system elevatorMod/PLCControllerSuite/__Logic/Task/Program/__Logic/XIC54/BlockEnableRead/__CoreLabelRead ==
  DataRead : DataStoreRead  DataStoreName=x_PLCLabel__s4_3653__Block_Enable
  Out1 : Outport  VectorParamsAs1DForOutWhenUnconnected=off
  wires:
  DataRead/1 -> Out1/1

== system elevatorMod/PLCControllerSuite/__Logic/Task/Program/__Logic/XIC54/Instruction_Enable/__CoreVarRead ==
  DataRead : DataStoreRead  DataStoreName=xxx_PLC_VAR_F3PBHold
  y : Outport  VectorParamsAs1DForOutWhenUnconnected=off
  wires:
  DataRead/1 -> y/1

== system elevatorMod/PLCControllerSuite/__Logic/Task/Program/__Logic/XIC54/RungInOverride/ForceRungInFalseRead ==
  __CoreLabelRead : Subsystem  Tag=CoreVarReadBlock  DisableCoverage=on  TreatAsAtomicUnit=on  mask{PLCBlockType=CoreLabelRead}
      mask init:
      | slplc.callbacks.initRoutineLabelRead(gcb);
      mask Help: web([docroot '/plccoder/ref/__corelabelread' '.html']);
      mask DialogControl PLCBlockTitle Prompt: Core Label Read
  Out1 : Outport  VectorParamsAs1DForOutWhenUnconnected=off
  wires:
  __CoreLabelRead/1(Out1) -> Out1/1

== system elevatorMod/PLCControllerSuite/__Logic/Task/Program/__Logic/XIC55/BlockEnableRead/__CoreLabelRead ==
  DataRead : DataStoreRead  DataStoreName=x_PLCLabel__s4_3653__Block_Enable
  Out1 : Outport  VectorParamsAs1DForOutWhenUnconnected=off
  wires:
  DataRead/1 -> Out1/1

== system elevatorMod/PLCControllerSuite/__Logic/Task/Program/__Logic/XIC55/Instruction_Enable/__CoreVarRead ==
  DataRead : DataStoreRead  DataStoreName=xxx_PLC_VAR_GOINGDN
  y : Outport  VectorParamsAs1DForOutWhenUnconnected=off
  wires:
  DataRead/1 -> y/1

== system elevatorMod/PLCControllerSuite/__Logic/Task/Program/__Logic/XIC55/RungInOverride/ForceRungInFalseRead ==
  __CoreLabelRead : Subsystem  Tag=CoreVarReadBlock  DisableCoverage=on  TreatAsAtomicUnit=on  mask{PLCBlockType=CoreLabelRead}
      mask init:
      | slplc.callbacks.initRoutineLabelRead(gcb);
      mask Help: web([docroot '/plccoder/ref/__corelabelread' '.html']);
      mask DialogControl PLCBlockTitle Prompt: Core Label Read
  Out1 : Outport  VectorParamsAs1DForOutWhenUnconnected=off
  wires:
  __CoreLabelRead/1(Out1) -> Out1/1

== system elevatorMod/PLCControllerSuite/__Logic/Task/Program/__Logic/XIC56/BlockEnableRead/__CoreLabelRead ==
  DataRead : DataStoreRead  DataStoreName=x_PLCLabel__s4_3653__Block_Enable
  Out1 : Outport  VectorParamsAs1DForOutWhenUnconnected=off
  wires:
  DataRead/1 -> Out1/1

== system elevatorMod/PLCControllerSuite/__Logic/Task/Program/__Logic/XIC56/Instruction_Enable/__CoreVarRead ==
  DataRead : DataStoreRead  DataStoreName=xxx_PLC_VAR_StartHold
  y : Outport  VectorParamsAs1DForOutWhenUnconnected=off
  wires:
  DataRead/1 -> y/1

== system elevatorMod/PLCControllerSuite/__Logic/Task/Program/__Logic/XIC56/RungInOverride/ForceRungInFalseRead ==
  __CoreLabelRead : Subsystem  Tag=CoreVarReadBlock  DisableCoverage=on  TreatAsAtomicUnit=on  mask{PLCBlockType=CoreLabelRead}
      mask init:
      | slplc.callbacks.initRoutineLabelRead(gcb);
      mask Help: web([docroot '/plccoder/ref/__corelabelread' '.html']);
      mask DialogControl PLCBlockTitle Prompt: Core Label Read
  Out1 : Outport  VectorParamsAs1DForOutWhenUnconnected=off
  wires:
  __CoreLabelRead/1(Out1) -> Out1/1

== system elevatorMod/PLCControllerSuite/__Logic/Task/Program/__Logic/XIC57/BlockEnableRead/__CoreLabelRead ==
  DataRead : DataStoreRead  DataStoreName=x_PLCLabel__s4_3653__Block_Enable
  Out1 : Outport  VectorParamsAs1DForOutWhenUnconnected=off
  wires:
  DataRead/1 -> Out1/1

== system elevatorMod/PLCControllerSuite/__Logic/Task/Program/__Logic/XIC57/Instruction_Enable/__CoreVarRead ==
  DataRead : DataStoreRead  DataStoreName=xxx_PLC_VAR_F1UpBHold
  y : Outport  VectorParamsAs1DForOutWhenUnconnected=off
  wires:
  DataRead/1 -> y/1

== system elevatorMod/PLCControllerSuite/__Logic/Task/Program/__Logic/XIC57/RungInOverride/ForceRungInFalseRead ==
  __CoreLabelRead : Subsystem  Tag=CoreVarReadBlock  DisableCoverage=on  TreatAsAtomicUnit=on  mask{PLCBlockType=CoreLabelRead}
      mask init:
      | slplc.callbacks.initRoutineLabelRead(gcb);
      mask Help: web([docroot '/plccoder/ref/__corelabelread' '.html']);
      mask DialogControl PLCBlockTitle Prompt: Core Label Read
  Out1 : Outport  VectorParamsAs1DForOutWhenUnconnected=off
  wires:
  __CoreLabelRead/1(Out1) -> Out1/1

== system elevatorMod/PLCControllerSuite/__Logic/Task/Program/__Logic/XIC58/BlockEnableRead/__CoreLabelRead ==
  DataRead : DataStoreRead  DataStoreName=x_PLCLabel__s4_3653__Block_Enable
  Out1 : Outport  VectorParamsAs1DForOutWhenUnconnected=off
  wires:
  DataRead/1 -> Out1/1

== system elevatorMod/PLCControllerSuite/__Logic/Task/Program/__Logic/XIC58/Instruction_Enable/__CoreVarRead ==
  DataRead : DataStoreRead  DataStoreName=xxx_PLC_VAR_StartHold
  y : Outport  VectorParamsAs1DForOutWhenUnconnected=off
  wires:
  DataRead/1 -> y/1

== system elevatorMod/PLCControllerSuite/__Logic/Task/Program/__Logic/XIC58/RungInOverride/ForceRungInFalseRead ==
  __CoreLabelRead : Subsystem  Tag=CoreVarReadBlock  DisableCoverage=on  TreatAsAtomicUnit=on  mask{PLCBlockType=CoreLabelRead}
      mask init:
      | slplc.callbacks.initRoutineLabelRead(gcb);
      mask Help: web([docroot '/plccoder/ref/__corelabelread' '.html']);
      mask DialogControl PLCBlockTitle Prompt: Core Label Read
  Out1 : Outport  VectorParamsAs1DForOutWhenUnconnected=off
  wires:
  __CoreLabelRead/1(Out1) -> Out1/1

== system elevatorMod/PLCControllerSuite/__Logic/Task/Program/__Logic/XIC59/BlockEnableRead/__CoreLabelRead ==
  DataRead : DataStoreRead  DataStoreName=x_PLCLabel__s4_3653__Block_Enable
  Out1 : Outport  VectorParamsAs1DForOutWhenUnconnected=off
  wires:
  DataRead/1 -> Out1/1

== system elevatorMod/PLCControllerSuite/__Logic/Task/Program/__Logic/XIC59/Instruction_Enable/__CoreVarRead ==
  DataRead : DataStoreRead  DataStoreName=xxx_PLC_VAR_StartHold
  y : Outport  VectorParamsAs1DForOutWhenUnconnected=off
  wires:
  DataRead/1 -> y/1

== system elevatorMod/PLCControllerSuite/__Logic/Task/Program/__Logic/XIC59/RungInOverride/ForceRungInFalseRead ==
  __CoreLabelRead : Subsystem  Tag=CoreVarReadBlock  DisableCoverage=on  TreatAsAtomicUnit=on  mask{PLCBlockType=CoreLabelRead}
      mask init:
      | slplc.callbacks.initRoutineLabelRead(gcb);
      mask Help: web([docroot '/plccoder/ref/__corelabelread' '.html']);
      mask DialogControl PLCBlockTitle Prompt: Core Label Read
  Out1 : Outport  VectorParamsAs1DForOutWhenUnconnected=off
  wires:
  __CoreLabelRead/1(Out1) -> Out1/1

== system elevatorMod/PLCControllerSuite/__Logic/Task/Program/__Logic/XIC6/BlockEnableRead/__CoreLabelRead ==
  DataRead : DataStoreRead  DataStoreName=x_PLCLabel__s4_3653__Block_Enable
  Out1 : Outport  VectorParamsAs1DForOutWhenUnconnected=off
  wires:
  DataRead/1 -> Out1/1

== system elevatorMod/PLCControllerSuite/__Logic/Task/Program/__Logic/XIC6/Instruction_Enable/__CoreVarRead ==
  DataRead : DataStoreRead  DataStoreName=xxx_PLC_VAR_StartHold
  y : Outport  VectorParamsAs1DForOutWhenUnconnected=off
  wires:
  DataRead/1 -> y/1

== system elevatorMod/PLCControllerSuite/__Logic/Task/Program/__Logic/XIC6/RungInOverride/ForceRungInFalseRead ==
  __CoreLabelRead : Subsystem  Tag=CoreVarReadBlock  DisableCoverage=on  TreatAsAtomicUnit=on  mask{PLCBlockType=CoreLabelRead}
      mask init:
      | slplc.callbacks.initRoutineLabelRead(gcb);
      mask Help: web([docroot '/plccoder/ref/__corelabelread' '.html']);
      mask DialogControl PLCBlockTitle Prompt: Core Label Read
  Out1 : Outport  VectorParamsAs1DForOutWhenUnconnected=off
  wires:
  __CoreLabelRead/1(Out1) -> Out1/1

== system elevatorMod/PLCControllerSuite/__Logic/Task/Program/__Logic/XIC60/BlockEnableRead/__CoreLabelRead ==
  DataRead : DataStoreRead  DataStoreName=x_PLCLabel__s4_3653__Block_Enable
  Out1 : Outport  VectorParamsAs1DForOutWhenUnconnected=off
  wires:
  DataRead/1 -> Out1/1

== system elevatorMod/PLCControllerSuite/__Logic/Task/Program/__Logic/XIC60/Instruction_Enable/__CoreVarRead ==
  DataRead : DataStoreRead  DataStoreName=xxx_PLC_VAR_S3L
  y : Outport  VectorParamsAs1DForOutWhenUnconnected=off
  wires:
  DataRead/1 -> y/1

== system elevatorMod/PLCControllerSuite/__Logic/Task/Program/__Logic/XIC60/RungInOverride/ForceRungInFalseRead ==
  __CoreLabelRead : Subsystem  Tag=CoreVarReadBlock  DisableCoverage=on  TreatAsAtomicUnit=on  mask{PLCBlockType=CoreLabelRead}
      mask init:
      | slplc.callbacks.initRoutineLabelRead(gcb);
      mask Help: web([docroot '/plccoder/ref/__corelabelread' '.html']);
      mask DialogControl PLCBlockTitle Prompt: Core Label Read
  Out1 : Outport  VectorParamsAs1DForOutWhenUnconnected=off
  wires:
  __CoreLabelRead/1(Out1) -> Out1/1

== system elevatorMod/PLCControllerSuite/__Logic/Task/Program/__Logic/XIC61/BlockEnableRead/__CoreLabelRead ==
  DataRead : DataStoreRead  DataStoreName=x_PLCLabel__s4_3653__Block_Enable
  Out1 : Outport  VectorParamsAs1DForOutWhenUnconnected=off
  wires:
  DataRead/1 -> Out1/1

== system elevatorMod/PLCControllerSuite/__Logic/Task/Program/__Logic/XIC61/Instruction_Enable/__CoreVarRead ==
  DataRead : DataStoreRead  DataStoreName=xxx_PLC_VAR_TempS3LUp
  y : Outport  VectorParamsAs1DForOutWhenUnconnected=off
  wires:
  DataRead/1 -> y/1

== system elevatorMod/PLCControllerSuite/__Logic/Task/Program/__Logic/XIC61/RungInOverride/ForceRungInFalseRead ==
  __CoreLabelRead : Subsystem  Tag=CoreVarReadBlock  DisableCoverage=on  TreatAsAtomicUnit=on  mask{PLCBlockType=CoreLabelRead}
      mask init:
      | slplc.callbacks.initRoutineLabelRead(gcb);
      mask Help: web([docroot '/plccoder/ref/__corelabelread' '.html']);
      mask DialogControl PLCBlockTitle Prompt: Core Label Read
  Out1 : Outport  VectorParamsAs1DForOutWhenUnconnected=off
  wires:
  __CoreLabelRead/1(Out1) -> Out1/1

== system elevatorMod/PLCControllerSuite/__Logic/Task/Program/__Logic/XIC62/BlockEnableRead/__CoreLabelRead ==
  DataRead : DataStoreRead  DataStoreName=x_PLCLabel__s4_3653__Block_Enable
  Out1 : Outport  VectorParamsAs1DForOutWhenUnconnected=off
  wires:
  DataRead/1 -> Out1/1

== system elevatorMod/PLCControllerSuite/__Logic/Task/Program/__Logic/XIC62/Instruction_Enable/__CoreVarRead ==
  DataRead : DataStoreRead  DataStoreName=xxx_PLC_VAR_S2H
  y : Outport  VectorParamsAs1DForOutWhenUnconnected=off
  wires:
  DataRead/1 -> y/1

== system elevatorMod/PLCControllerSuite/__Logic/Task/Program/__Logic/XIC62/RungInOverride/ForceRungInFalseRead ==
  __CoreLabelRead : Subsystem  Tag=CoreVarReadBlock  DisableCoverage=on  TreatAsAtomicUnit=on  mask{PLCBlockType=CoreLabelRead}
      mask init:
      | slplc.callbacks.initRoutineLabelRead(gcb);
      mask Help: web([docroot '/plccoder/ref/__corelabelread' '.html']);
      mask DialogControl PLCBlockTitle Prompt: Core Label Read
  Out1 : Outport  VectorParamsAs1DForOutWhenUnconnected=off
  wires:
  __CoreLabelRead/1(Out1) -> Out1/1

== system elevatorMod/PLCControllerSuite/__Logic/Task/Program/__Logic/XIC63/BlockEnableRead/__CoreLabelRead ==
  DataRead : DataStoreRead  DataStoreName=x_PLCLabel__s4_3653__Block_Enable
  Out1 : Outport  VectorParamsAs1DForOutWhenUnconnected=off
  wires:
  DataRead/1 -> Out1/1

== system elevatorMod/PLCControllerSuite/__Logic/Task/Program/__Logic/XIC63/Instruction_Enable/__CoreVarRead ==
  DataRead : DataStoreRead  DataStoreName=xxx_PLC_VAR_TempS2HDown
  y : Outport  VectorParamsAs1DForOutWhenUnconnected=off
  wires:
  DataRead/1 -> y/1

== system elevatorMod/PLCControllerSuite/__Logic/Task/Program/__Logic/XIC63/RungInOverride/ForceRungInFalseRead ==
  __CoreLabelRead : Subsystem  Tag=CoreVarReadBlock  DisableCoverage=on  TreatAsAtomicUnit=on  mask{PLCBlockType=CoreLabelRead}
      mask init:
      | slplc.callbacks.initRoutineLabelRead(gcb);
      mask Help: web([docroot '/plccoder/ref/__corelabelread' '.html']);
      mask DialogControl PLCBlockTitle Prompt: Core Label Read
  Out1 : Outport  VectorParamsAs1DForOutWhenUnconnected=off
  wires:
  __CoreLabelRead/1(Out1) -> Out1/1

== system elevatorMod/PLCControllerSuite/__Logic/Task/Program/__Logic/XIC64/BlockEnableRead/__CoreLabelRead ==
  DataRead : DataStoreRead  DataStoreName=x_PLCLabel__s4_3653__Block_Enable
  Out1 : Outport  VectorParamsAs1DForOutWhenUnconnected=off
  wires:
  DataRead/1 -> Out1/1

== system elevatorMod/PLCControllerSuite/__Logic/Task/Program/__Logic/XIC64/Instruction_Enable/__CoreVarRead ==
  DataRead : DataStoreRead  DataStoreName=xxx_PLC_VAR_S2L
  y : Outport  VectorParamsAs1DForOutWhenUnconnected=off
  wires:
  DataRead/1 -> y/1

== system elevatorMod/PLCControllerSuite/__Logic/Task/Program/__Logic/XIC64/RungInOverride/ForceRungInFalseRead ==
  __CoreLabelRead : Subsystem  Tag=CoreVarReadBlock  DisableCoverage=on  TreatAsAtomicUnit=on  mask{PLCBlockType=CoreLabelRead}
      mask init:
      | slplc.callbacks.initRoutineLabelRead(gcb);
      mask Help: web([docroot '/plccoder/ref/__corelabelread' '.html']);
      mask DialogControl PLCBlockTitle Prompt: Core Label Read
  Out1 : Outport  VectorParamsAs1DForOutWhenUnconnected=off
  wires:
  __CoreLabelRead/1(Out1) -> Out1/1

== system elevatorMod/PLCControllerSuite/__Logic/Task/Program/__Logic/XIC65/BlockEnableRead/__CoreLabelRead ==
  DataRead : DataStoreRead  DataStoreName=x_PLCLabel__s4_3653__Block_Enable
  Out1 : Outport  VectorParamsAs1DForOutWhenUnconnected=off
  wires:
  DataRead/1 -> Out1/1

== system elevatorMod/PLCControllerSuite/__Logic/Task/Program/__Logic/XIC65/Instruction_Enable/__CoreVarRead ==
  DataRead : DataStoreRead  DataStoreName=xxx_PLC_VAR_TempS2LDown
  y : Outport  VectorParamsAs1DForOutWhenUnconnected=off
  wires:
  DataRead/1 -> y/1

== system elevatorMod/PLCControllerSuite/__Logic/Task/Program/__Logic/XIC65/RungInOverride/ForceRungInFalseRead ==
  __CoreLabelRead : Subsystem  Tag=CoreVarReadBlock  DisableCoverage=on  TreatAsAtomicUnit=on  mask{PLCBlockType=CoreLabelRead}
      mask init:
      | slplc.callbacks.initRoutineLabelRead(gcb);
      mask Help: web([docroot '/plccoder/ref/__corelabelread' '.html']);
      mask DialogControl PLCBlockTitle Prompt: Core Label Read
  Out1 : Outport  VectorParamsAs1DForOutWhenUnconnected=off
  wires:
  __CoreLabelRead/1(Out1) -> Out1/1

== system elevatorMod/PLCControllerSuite/__Logic/Task/Program/__Logic/XIC66/BlockEnableRead/__CoreLabelRead ==
  DataRead : DataStoreRead  DataStoreName=x_PLCLabel__s4_3653__Block_Enable
  Out1 : Outport  VectorParamsAs1DForOutWhenUnconnected=off
  wires:
  DataRead/1 -> Out1/1

== system elevatorMod/PLCControllerSuite/__Logic/Task/Program/__Logic/XIC66/Instruction_Enable/__CoreVarRead ==
  DataRead : DataStoreRead  DataStoreName=xxx_PLC_VAR_S1H
  y : Outport  VectorParamsAs1DForOutWhenUnconnected=off
  wires:
  DataRead/1 -> y/1

== system elevatorMod/PLCControllerSuite/__Logic/Task/Program/__Logic/XIC66/RungInOverride/ForceRungInFalseRead ==
  __CoreLabelRead : Subsystem  Tag=CoreVarReadBlock  DisableCoverage=on  TreatAsAtomicUnit=on  mask{PLCBlockType=CoreLabelRead}
      mask init:
      | slplc.callbacks.initRoutineLabelRead(gcb);
      mask Help: web([docroot '/plccoder/ref/__corelabelread' '.html']);
      mask DialogControl PLCBlockTitle Prompt: Core Label Read
  Out1 : Outport  VectorParamsAs1DForOutWhenUnconnected=off
  wires:
  __CoreLabelRead/1(Out1) -> Out1/1

== system elevatorMod/PLCControllerSuite/__Logic/Task/Program/__Logic/XIC67/BlockEnableRead/__CoreLabelRead ==
  DataRead : DataStoreRead  DataStoreName=x_PLCLabel__s4_3653__Block_Enable
  Out1 : Outport  VectorParamsAs1DForOutWhenUnconnected=off
  wires:
  DataRead/1 -> Out1/1

== system elevatorMod/PLCControllerSuite/__Logic/Task/Program/__Logic/XIC67/Instruction_Enable/__CoreVarRead ==
  DataRead : DataStoreRead  DataStoreName=xxx_PLC_VAR_TempS1HDown
  y : Outport  VectorParamsAs1DForOutWhenUnconnected=off
  wires:
  DataRead/1 -> y/1

== system elevatorMod/PLCControllerSuite/__Logic/Task/Program/__Logic/XIC67/RungInOverride/ForceRungInFalseRead ==
  __CoreLabelRead : Subsystem  Tag=CoreVarReadBlock  DisableCoverage=on  TreatAsAtomicUnit=on  mask{PLCBlockType=CoreLabelRead}
      mask init:
      | slplc.callbacks.initRoutineLabelRead(gcb);
      mask Help: web([docroot '/plccoder/ref/__corelabelread' '.html']);
      mask DialogControl PLCBlockTitle Prompt: Core Label Read
  Out1 : Outport  VectorParamsAs1DForOutWhenUnconnected=off
  wires:
  __CoreLabelRead/1(Out1) -> Out1/1

== system elevatorMod/PLCControllerSuite/__Logic/Task/Program/__Logic/XIC68/BlockEnableRead/__CoreLabelRead ==
  DataRead : DataStoreRead  DataStoreName=x_PLCLabel__s4_3653__Block_Enable
  Out1 : Outport  VectorParamsAs1DForOutWhenUnconnected=off
  wires:
  DataRead/1 -> Out1/1

== system elevatorMod/PLCControllerSuite/__Logic/Task/Program/__Logic/XIC68/Instruction_Enable/__CoreVarRead ==
  DataRead : DataStoreRead  DataStoreName=xxx_PLC_VAR_StartHold
  y : Outport  VectorParamsAs1DForOutWhenUnconnected=off
  wires:
  DataRead/1 -> y/1

== system elevatorMod/PLCControllerSuite/__Logic/Task/Program/__Logic/XIC68/RungInOverride/ForceRungInFalseRead ==
  __CoreLabelRead : Subsystem  Tag=CoreVarReadBlock  DisableCoverage=on  TreatAsAtomicUnit=on  mask{PLCBlockType=CoreLabelRead}
      mask init:
      | slplc.callbacks.initRoutineLabelRead(gcb);
      mask Help: web([docroot '/plccoder/ref/__corelabelread' '.html']);
      mask DialogControl PLCBlockTitle Prompt: Core Label Read
  Out1 : Outport  VectorParamsAs1DForOutWhenUnconnected=off
  wires:
  __CoreLabelRead/1(Out1) -> Out1/1

== system elevatorMod/PLCControllerSuite/__Logic/Task/Program/__Logic/XIC69/BlockEnableRead/__CoreLabelRead ==
  DataRead : DataStoreRead  DataStoreName=x_PLCLabel__s4_3653__Block_Enable
  Out1 : Outport  VectorParamsAs1DForOutWhenUnconnected=off
  wires:
  DataRead/1 -> Out1/1

== system elevatorMod/PLCControllerSuite/__Logic/Task/Program/__Logic/XIC69/Instruction_Enable/__CoreVarRead ==
  DataRead : DataStoreRead  DataStoreName=xxx_PLC_VAR_StartHold
  y : Outport  VectorParamsAs1DForOutWhenUnconnected=off
  wires:
  DataRead/1 -> y/1

== system elevatorMod/PLCControllerSuite/__Logic/Task/Program/__Logic/XIC69/RungInOverride/ForceRungInFalseRead ==
  __CoreLabelRead : Subsystem  Tag=CoreVarReadBlock  DisableCoverage=on  TreatAsAtomicUnit=on  mask{PLCBlockType=CoreLabelRead}
      mask init:
      | slplc.callbacks.initRoutineLabelRead(gcb);
      mask Help: web([docroot '/plccoder/ref/__corelabelread' '.html']);
      mask DialogControl PLCBlockTitle Prompt: Core Label Read
  Out1 : Outport  VectorParamsAs1DForOutWhenUnconnected=off
  wires:
  __CoreLabelRead/1(Out1) -> Out1/1

== system elevatorMod/PLCControllerSuite/__Logic/Task/Program/__Logic/XIC7/BlockEnableRead/__CoreLabelRead ==
  DataRead : DataStoreRead  DataStoreName=x_PLCLabel__s4_3653__Block_Enable
  Out1 : Outport  VectorParamsAs1DForOutWhenUnconnected=off
  wires:
  DataRead/1 -> Out1/1

== system elevatorMod/PLCControllerSuite/__Logic/Task/Program/__Logic/XIC7/Instruction_Enable/__CoreVarRead ==
  DataRead : DataStoreRead  DataStoreName=xxx_PLC_VAR_F2PB
  y : Outport  VectorParamsAs1DForOutWhenUnconnected=off
  wires:
  DataRead/1 -> y/1

== system elevatorMod/PLCControllerSuite/__Logic/Task/Program/__Logic/XIC7/RungInOverride/ForceRungInFalseRead ==
  __CoreLabelRead : Subsystem  Tag=CoreVarReadBlock  DisableCoverage=on  TreatAsAtomicUnit=on  mask{PLCBlockType=CoreLabelRead}
      mask init:
      | slplc.callbacks.initRoutineLabelRead(gcb);
      mask Help: web([docroot '/plccoder/ref/__corelabelread' '.html']);
      mask DialogControl PLCBlockTitle Prompt: Core Label Read
  Out1 : Outport  VectorParamsAs1DForOutWhenUnconnected=off
  wires:
  __CoreLabelRead/1(Out1) -> Out1/1

== system elevatorMod/PLCControllerSuite/__Logic/Task/Program/__Logic/XIC70/BlockEnableRead/__CoreLabelRead ==
  DataRead : DataStoreRead  DataStoreName=x_PLCLabel__s4_3653__Block_Enable
  Out1 : Outport  VectorParamsAs1DForOutWhenUnconnected=off
  wires:
  DataRead/1 -> Out1/1

== system elevatorMod/PLCControllerSuite/__Logic/Task/Program/__Logic/XIC70/Instruction_Enable/__CoreVarRead ==
  DataRead : DataStoreRead  DataStoreName=xxx_PLC_VAR_TempS2HUp
  y : Outport  VectorParamsAs1DForOutWhenUnconnected=off
  wires:
  DataRead/1 -> y/1
